simulink model "mcb_pmsm_foc_hall_f28069m"  (R2023b)
settings: Solver=FixedStepDiscrete  StartTime=0.0  StopTime=8  RelTol=1e-3  EnableMultiTasking=on
InitFcn:
  | mcb_pmsm_foc_hall_f28069m_data;
values from neighbouring files (symbols this model uses):
  inverter = mcb_SetInverterParameters('DRV8312-C2-KIT')    [mcb_pmsm_foc_hall_f28069m_data.m]    (also in mcb_pmsm_foc_hall_f28379d_data.m = mcb_updateInverterParameters(pmsm,inverter,target))
  PI_params = mcb_SetControllerParameters(pmsm,inverter,PU_System,T_pwm,Ts,Ts_speed)    [mcb_pmsm_foc_hall_f28069m_data.m]    (also in mcb_pmsm_foc_hall_f28379d_data.m)
  pmsm = mcb_SetPMSMMotorParameters('BLY171D')    [mcb_pmsm_foc_hall_f28069m_data.m]    (also in mcb_pmsm_foc_hall_f28379d_data.m = mcb_SetPMSMMotorParameters("custom"))
  target = mcb_SetProcessorDetails('F28069M',PWM_frequency)    [mcb_pmsm_foc_hall_f28069m_data.m]    (also in mcb_pmsm_foc_hall_f28379d_data.m = mcb_SetProcessorDetails('F28379D',PWM_frequency))
  Ts = T_pwm    (= 5e-05)    [mcb_pmsm_foc_hall_f28069m_data.m]    (also in mcb_pmsm_foc_hall_f28379d_data.m = 6.25e-05)
  Ts_motor = T_pwm/2    (= 2.5e-05)    [mcb_pmsm_foc_hall_f28069m_data.m]    (also in mcb_pmsm_foc_hall_f28379d_data.m = 3.125e-05)
  Ts_simulink = T_pwm/2    (= 2.5e-05)    [mcb_pmsm_foc_hall_f28069m_data.m]    (also in mcb_pmsm_foc_hall_f28379d_data.m = 3.125e-05)
  Ts_speed = 10*Ts    (= 0.0005)    [mcb_pmsm_foc_hall_f28069m_data.m]    (also in mcb_pmsm_foc_hall_f28379d_data.m = 0.000625)
undefined symbols (not defined in the file or in its folder): Down, GPTRIP1SEL, GPTRIP2SEL, TZ1, TZ2, Up
libraries: simulink x14, mcbcontrolslib x9, mcbpositiondecoderlib x7, idelinklib_common x6, c2802xlib x5, c280xlib x5, svdschedulerlib x5, slpidlib x3, c2806xlib x3, svdutilitieslib x2, mcbplantlib x1, autolibpmsmexterior x1
(part 1 of 3)
settings Model: Creator=The MathWorks, Inc.  LastModifiedBy=The MathWorks, Inc.
settings SolverCC: AlgebraicLoopSolver=TrustRegion  AutoInsertRateTranBlk=on
settings DataIOCC: LimitDataPoints=on  SaveFormat=Array  SaveOutput=off  SaveTime=off  ReturnWorkspaceOutputs=off
settings OptimizationCC: DefaultParameterBehavior=Inlined  InlineInvariantSignals=on  OptimizeBlockIOStorage=off  BufferReuse=off  ReuseModelBlockBuffer=off  GlobalBufferReuse=off  ExpressionFolding=off  ExpressionDepthLimit=2147483647  LocalBlockOutputs=off  InitFltsAndDblsToZero=on  NoFixptDivByZeroProtection=on  EfficientFloat2IntCast=on  EfficientMapNaN2IntZero=off  LifeSpan=inf  MaxStackSize=64  OptimizeDataStoreBuffers=off  BusAssignmentInplaceUpdate=off  EfficientTunableParamExpr=on
settings DebuggingCC: AlgebraicLoopMsg=error  ArtificialAlgebraicLoopMsg=error  CheckSSInitialOutputMsg=off  MergeDetectMultiDrivingBlocksExec=none  SolverPrmCheckMsg=warning  InheritedTsInSrcMsg=none  MultiTaskDSMMsg=none  MultiTaskCondExecSysMsg=none  TasksWithSamePriorityMsg=none  SigSpecEnsureSampleTimeMsg=none  ParameterPrecisionLossMsg=none  ParameterTunabilityLossMsg=error  FcnCallInpInsideContextMsg=warning  UnconnectedInputMsg=warning  UnconnectedOutputMsg=warning  UnconnectedLineMsg=warning  AllowSymbolicDim=off  StateNameClashWarn=warning  SFUnexpectedBacktrackingDiag=warning  SFNoUnconditionalDefaultTransitionDiag=warning  SFExecutionAtInitializationDiag=none  ArithmeticOperatorsInVariantConditions=warning
settings HardwareCC: ProdBitPerChar=16  ProdBitPerInt=16  ProdBitPerPointer=32  ProdBitPerSizeT=32  ProdBitPerPtrDiffT=32  ProdLargestAtomicInteger=Integer  ProdLargestAtomicFloat=None  ProdWordSize=16  ProdLongLongMode=on  ProdHWDeviceType=Texas Instruments->C2000  TargetBitPerChar=16  TargetBitPerInt=16  TargetBitPerPointer=16  TargetLargestAtomicInteger=Integer  TargetIntDivRoundTo=Zero  TargetEndianess=LittleEndian  TargetWordSize=16  TargetHWDeviceType=Texas Instruments->C2000  ProdEqTarget=off
settings ModelReferenceCC: EnableRefExpFcnMdlSchedulingChecks=on  PropagateSignalLabelsOutOfModel=off
settings SFSimCC: SimUseLocalCustomCode=off  MATLABDynamicMemAlloc=off
settings RTWCC: Description=Embedded Coder  SystemTargetFile=ert.tlc  HardwareBoard=TI Piccolo F2806x  TemplateMakefile=ert_default_tmf  PostCodeGenCommand=; codertarget.postCodeGenHookCommand(h)  GenerateReport=on  RTWUseLocalCustomCode=off  Toolchain=Texas Instruments Code Composer Studio (C2000)  IncludeHyperlinkInReport=on  GenerateTraceInfo=on  GenerateTraceReport=on  GenerateTraceReportSl=on  GenerateTraceReportSf=on  GenerateTraceReportEml=on  DLArmComputeVersion=19.05
settings CodeAppCC: IgnoreCustomStorageClasses=off  CustomSymbolStrType=$N$R$M  StateflowObjectComments=on  InternalIdentifier=Classic
settings ERTTargetCC: TargetFcnLib=ansi_tfl_tmw_new.mat  CodeReplacementLibrary=TI C28x  MultiwordLength=2048  ParMdlRefBuildCompliant=off  CompOptLevelCompliant=off  ConcurrentExecutionCompliant=off  CPPClassGenCompliant=off  ExtModeStaticAllocSize=2048  ExtModeMexFile=TIC2000ExternalModeOpen  ExtModeIntrfLevel=Level2 - Open  InlinedParameterPlacement=NonHierarchical  ConvertIfToSwitch=off  SuppressUnreachableDefaultCases=off  MemSecPackage=tic2000demospkg
settings ConfigComp: CovMetricSettings=dw  CovSaveCumulativeToWorkspaceVar=on  CovSaveSingleToWorkspaceVar=on  CovExternalEMLEnable=off  CovSFcnEnable=off

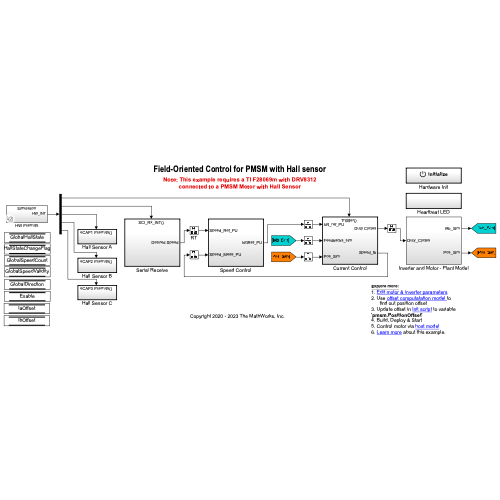
[thumbnail: Simulink's stored preview of the top-level diagram]
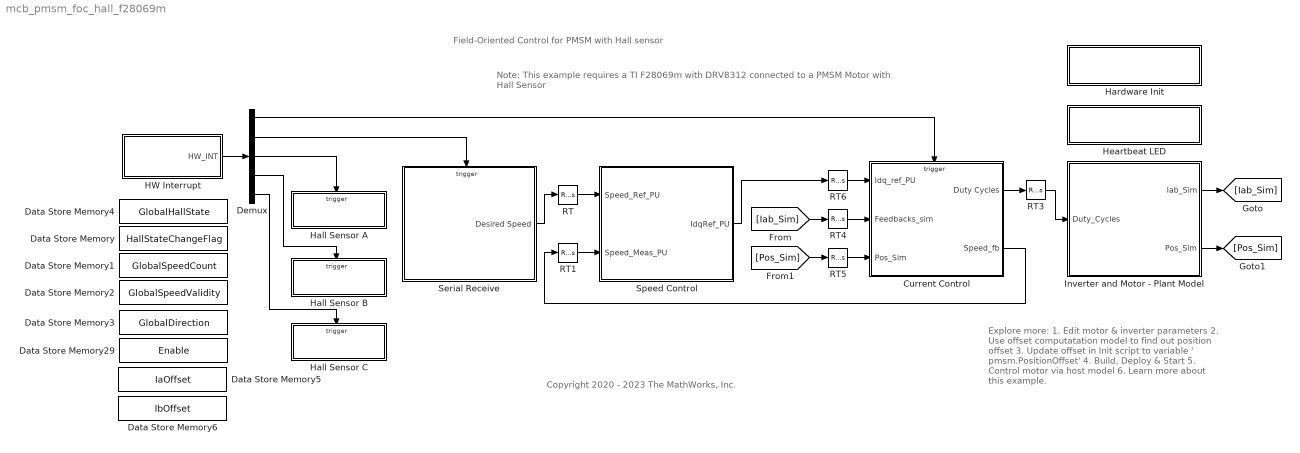
== system mcb_pmsm_foc_hall_f28069m ==
  note: Copyright 2020 - 2023 The MathWorks, Inc.
  note: Field-Oriented Control for PMSM with Hall sensor
  note: Note: This example requires a TI F28069m with DRV8312
      | connected to a PMSM Motor with Hall Sensor
  note: Explore more:
      | 1. Edit motor & inverter parameters
      | 2. Use offset computatation model to
      | find out position offset
      | 3. Update offset in Init script to variable ' pmsm.PositionOffset'
      | 4. Build, Deploy & Start
      | 5. Control motor via host model
      | 6. Learn more about this example.
  Current Control : Subsystem
      settings: RTWSystemCode=Nonreusable function
  Data Store Memory : DataStoreMemory  DataStoreName=HallStateChangeFlag  ShowAdditionalParam=off
  Data Store Memory1 : DataStoreMemory  DataStoreName=GlobalSpeedCount  ShowAdditionalParam=off
  Data Store Memory2 : DataStoreMemory  DataStoreName=GlobalSpeedValidity  ShowAdditionalParam=off
  Data Store Memory29 : DataStoreMemory  DataStoreName=Enable  InitialValue=1  ShowAdditionalParam=off  OutDataTypeStr=boolean
  Data Store Memory3 : DataStoreMemory  DataStoreName=GlobalDirection  ShowAdditionalParam=off
  Data Store Memory4 : DataStoreMemory  DataStoreName=GlobalHallState  ShowAdditionalParam=off  OutDataTypeStr=uint32
  Data Store Memory5 : DataStoreMemory  DataStoreName=IaOffset  InitialValue=inverter.CtSensAOffset  ShowAdditionalParam=off
  Data Store Memory6 : DataStoreMemory  DataStoreName=IbOffset  InitialValue=inverter.CtSensBOffset  ShowAdditionalParam=off
  Demux : Demux  Outputs=5
  HW Interrupt : Subsystem  Variant=on  VariantControlMode=sim codegen switching
  Hall Sensor A : Subsystem
  Hall Sensor B : Subsystem
  Hall Sensor C : Subsystem
  Hardware Init : Subsystem  TreatAsAtomicUnit=on
  Heartbeat LED : Subsystem  TreatAsAtomicUnit=on
  Inverter and Motor - Plant Model : Subsystem
  RT{,3..6} (5 alike) : RateTransition  Deterministic=off
  RT1 : RateTransition  Deterministic=off  OutPortSampleTime=Ts_speed
  Serial Receive : Subsystem  SystemSampleTime=1e-3
  Speed Control : Subsystem  TreatAsAtomicUnit=on  SystemSampleTime=Ts_speed
  wires:
  [Iab_Sim] -> RT4/1
  RT1/1 -> Speed Control/2(Speed_Meas_PU)
  [Pos_Sim] -> RT5/1
  Speed Control/1(IdqRef_PU) -> RT6/1
  Inverter and Motor - Plant Model/1(Iab_Sim) -> [Iab_Sim]
  RT/1 -> Speed Control/1(Speed_Ref_PU)
  Demux/3 -> Hall Sensor A/Trigger
  Demux/5 -> Hall Sensor C/Trigger
  RT6/1 -> Current Control/1(Idq_ref_PU)
  HW Interrupt/1(HW_INT) -> Demux/1
  Demux/1 -> Current Control/Trigger
  RT3/1 -> Inverter and Motor - Plant Model/1(Duty_Cycles)
  Demux/2 -> Serial Receive/Trigger
  RT4/1 -> Current Control/2(Feedbacks_sim)
  Serial Receive/1(Desired Speed) -> RT/1
  Current Control/1(Duty Cycles) -> RT3/1
  Inverter and Motor - Plant Model/2(Pos_Sim) -> [Pos_Sim]
  Demux/4 -> Hall Sensor B/Trigger
  RT5/1 -> Current Control/3(Pos_Sim)
  Current Control/2(Speed_fb) -> RT1/1

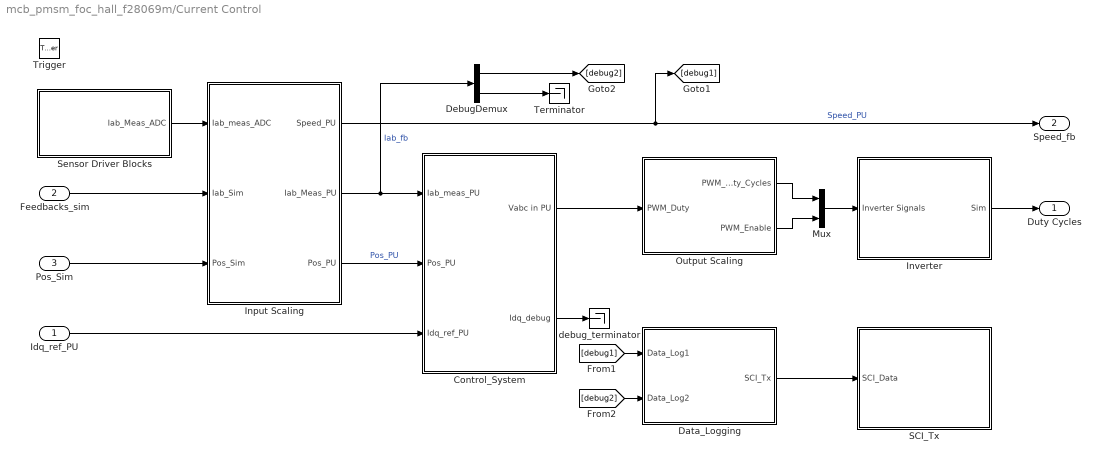
== system mcb_pmsm_foc_hall_f28069m/Current Control ==
  Idq_ref_PU : Inport
  Feedbacks_sim : Inport  Port=2
  Pos_Sim : Inport  Port=3
  Trigger : TriggerPort  TriggerType=function-call  VariantControl=Variant
  Control_System : Subsystem
  Data_Logging : Subsystem
  DebugDemux : Demux  Outputs=2
  Input Scaling : Subsystem  Variant=on  VariantControlMode=sim codegen switching  VariantControl=Variant1  PropagateVariantConditions=on
  Inverter : Subsystem  Variant=on  VariantControlMode=sim codegen switching
  Mux : Mux  Inputs=2
  Output Scaling : Subsystem
  SCI_Tx : Subsystem  Variant=on  VariantControlMode=sim codegen switching
  Sensor Driver Blocks : Subsystem  Variant=on  VariantControlMode=sim codegen switching
  Terminator : Terminator
  debug_terminator : Terminator
  Duty Cycles : Outport  InitialOutput=0  VectorParamsAs1DForOutWhenUnconnected=off
  Speed_fb : Outport  Port=2  InitialOutput=0  VectorParamsAs1DForOutWhenUnconnected=off
  wires:
  Sensor Driver Blocks/1(Iab_Meas_ADC) -> Input Scaling/1(Iab_meas_ADC)
  Control_System/1(Vabc in PU) -> Output Scaling/1(PWM_Duty)
  Input Scaling/3(Pos_PU) -> Control_System/2(Pos_PU)  "Pos_PU"
  Idq_ref_PU/1 -> Control_System/3(Idq_ref_PU)
  Input Scaling/2(Iab_Meas_PU) -> DebugDemux/1, Control_System/1(Iab_meas_PU)  "Iab_fb"
  Input Scaling/1(Speed_PU) -> [debug1], Speed_fb/1  "Speed_PU"
  Pos_Sim/1 -> Input Scaling/3(Pos_Sim)
  Feedbacks_sim/1 -> Input Scaling/2(Iab_Sim)
  Mux/1 -> Inverter/1(Inverter Signals)
  Output Scaling/1(PWM_Duty_Cycles) -> Mux/1
  Output Scaling/2(PWM_Enable) -> Mux/2
  Inverter/1(Sim) -> Duty Cycles/1
  [debug2] -> Data_Logging/2(Data_Log2)
  [debug1] -> Data_Logging/1(Data_Log1)
  DebugDemux/1 -> [debug2]
  DebugDemux/2 -> Terminator/1
  Control_System/2(Idq_debug) -> debug_terminator/1
  Data_Logging/1(SCI_Tx) -> SCI_Tx/1(SCI_Data)

== system mcb_pmsm_foc_hall_f28069m/HW Interrupt ==
  Code Generation : Subsystem  VariantControl=(codegen)
  Simulation : Subsystem  VariantControl=(sim)
  HW_INT : Outport  VectorParamsAs1DForOutWhenUnconnected=off  OutputFunctionCall=on

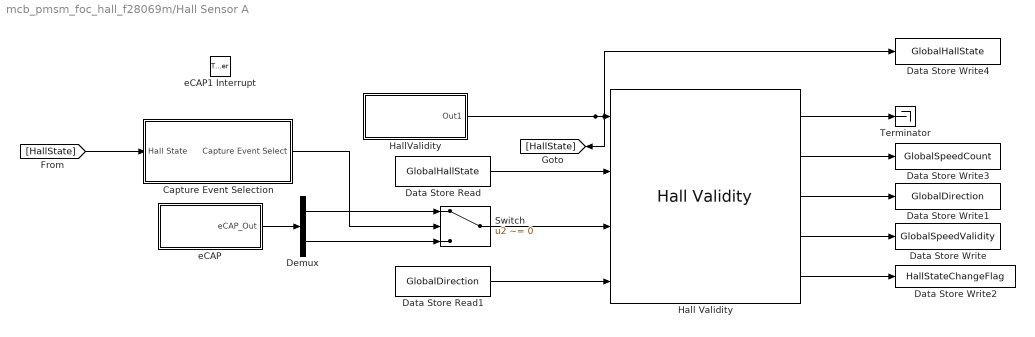
== system mcb_pmsm_foc_hall_f28069m/Hall Sensor A ==
  eCAP1 Interrupt : TriggerPort  TriggerType=function-call  VariantControl=Variant
  Capture Event Selection : Subsystem
  Data Store Read : DataStoreRead  Priority=1  DataStoreName=GlobalHallState  IndexOptions=Index vector (dialog)  Indices=1  OutputSizes=1
  Data Store Read1 : DataStoreRead  DataStoreName=GlobalDirection  IndexOptions=Index vector (dialog)  Indices=1  OutputSizes=1
  Data Store Write : DataStoreWrite  DataStoreName=GlobalSpeedValidity  IndexOptions=Index vector (dialog)  Indices=1  OutputSizes=1
  Data Store Write1 : DataStoreWrite  DataStoreName=GlobalDirection  IndexOptions=Index vector (dialog)  Indices=1  OutputSizes=1
  Data Store Write2 : DataStoreWrite  DataStoreName=HallStateChangeFlag  IndexOptions=Index vector (dialog)  Indices=1  OutputSizes=1
  Data Store Write3 : DataStoreWrite  DataStoreName=GlobalSpeedCount  IndexOptions=Index vector (dialog)  Indices=1  OutputSizes=1
  Data Store Write4 : DataStoreWrite  Priority=2  DataStoreName=GlobalHallState  IndexOptions=Index vector (dialog)  Indices=1  OutputSizes=1
  Demux : Demux  Outputs=2
  Hall Validity : mcbpositiondecoderlib/Hall Validity  hallSequence=ABC  sequence=[5,4,6,2,3,1]  CounterSize=32 bits
  HallValidity : Subsystem  Variant=on  VariantControlMode=sim codegen switching
  Switch : Switch  Criteria=u2 ~= 0  SaturateOnIntegerOverflow=off  InputSameDT=off
  Terminator : Terminator
  eCAP : Subsystem  Variant=on  VariantControlMode=sim codegen switching
  wires:
  Hall Validity/3 -> Data Store Write1/1
  Hall Validity/5 -> Data Store Write2/1
  Hall Validity/4 -> Data Store Write/1
  Data Store Read/1 -> Hall Validity/2
  Data Store Read1/1 -> Hall Validity/4
  Switch/1 -> Hall Validity/3
  Hall Validity/2 -> Data Store Write3/1
  Demux/2 -> Switch/3
  Demux/1 -> Switch/1
  Hall Validity/1 -> Terminator/1
  Capture Event Selection/1(Capture Event Select) -> Switch/2
  [HallState] -> Capture Event Selection/1(Hall State)
  eCAP/1(eCAP_Out) -> Demux/1
  HallValidity/1(Out1) -> [HallState], Data Store Write4/1, Hall Validity/1

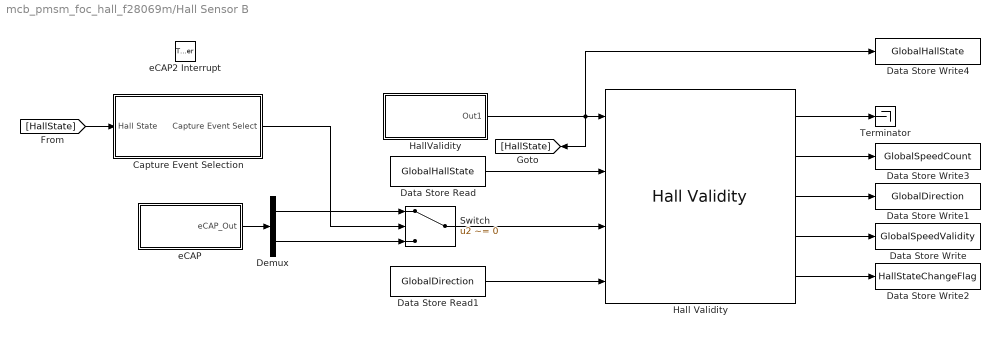
== system mcb_pmsm_foc_hall_f28069m/Hall Sensor B ==
  eCAP2 Interrupt : TriggerPort  TriggerType=function-call  VariantControl=Variant
  Capture Event Selection : Subsystem
  Data Store Read : DataStoreRead  Priority=1  DataStoreName=GlobalHallState  IndexOptions=Index vector (dialog)  Indices=1  OutputSizes=1
  Data Store Read1 : DataStoreRead  DataStoreName=GlobalDirection  IndexOptions=Index vector (dialog)  Indices=1  OutputSizes=1
  Data Store Write : DataStoreWrite  DataStoreName=GlobalSpeedValidity  IndexOptions=Index vector (dialog)  Indices=1  OutputSizes=1
  Data Store Write1 : DataStoreWrite  DataStoreName=GlobalDirection  IndexOptions=Index vector (dialog)  Indices=1  OutputSizes=1
  Data Store Write2 : DataStoreWrite  DataStoreName=HallStateChangeFlag  IndexOptions=Index vector (dialog)  Indices=1  OutputSizes=1
  Data Store Write3 : DataStoreWrite  DataStoreName=GlobalSpeedCount  IndexOptions=Index vector (dialog)  Indices=1  OutputSizes=1
  Data Store Write4 : DataStoreWrite  Priority=2  DataStoreName=GlobalHallState  IndexOptions=Index vector (dialog)  Indices=1  OutputSizes=1
  Demux : Demux  Outputs=2
  Hall Validity : mcbpositiondecoderlib/Hall Validity  hallSequence=ABC  sequence=[5,4,6,2,3,1]  CounterSize=32 bits
  HallValidity : Subsystem  Variant=on  VariantControlMode=sim codegen switching
  Switch : Switch  Criteria=u2 ~= 0  Threshold=3  SaturateOnIntegerOverflow=off  InputSameDT=off
  Terminator : Terminator
  eCAP : Subsystem  Variant=on  VariantControlMode=sim codegen switching
  wires:
  Hall Validity/3 -> Data Store Write1/1
  Hall Validity/5 -> Data Store Write2/1
  Hall Validity/4 -> Data Store Write/1
  Data Store Read1/1 -> Hall Validity/4
  Hall Validity/2 -> Data Store Write3/1
  Data Store Read/1 -> Hall Validity/2
  Demux/1 -> Switch/1
  Demux/2 -> Switch/3
  eCAP/1(eCAP_Out) -> Demux/1
  Switch/1 -> Hall Validity/3
  Hall Validity/1 -> Terminator/1
  [HallState] -> Capture Event Selection/1(Hall State)
  Capture Event Selection/1(Capture Event Select) -> Switch/2
  HallValidity/1(Out1) -> Data Store Write4/1, Hall Validity/1, [HallState]

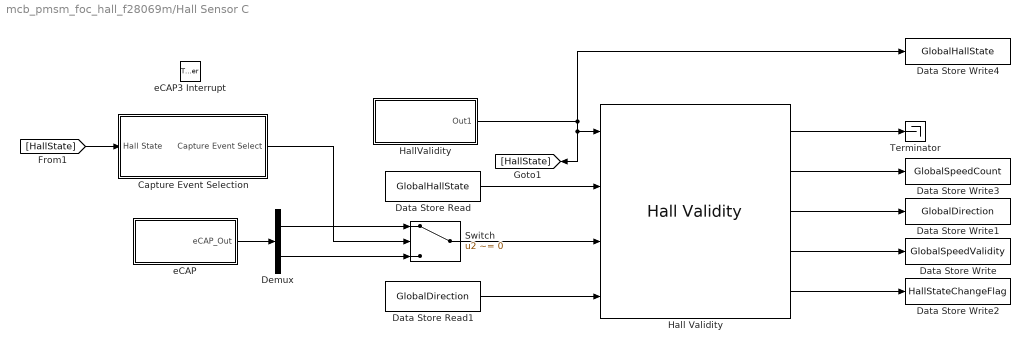
== system mcb_pmsm_foc_hall_f28069m/Hall Sensor C ==
  eCAP3 Interrupt : TriggerPort  TriggerType=function-call  VariantControl=Variant
  Capture Event Selection : Subsystem
  Data Store Read : DataStoreRead  Priority=1  DataStoreName=GlobalHallState  IndexOptions=Index vector (dialog)  Indices=1  OutputSizes=1
  Data Store Read1 : DataStoreRead  DataStoreName=GlobalDirection  IndexOptions=Index vector (dialog)  Indices=1  OutputSizes=1
  Data Store Write : DataStoreWrite  DataStoreName=GlobalSpeedValidity  IndexOptions=Index vector (dialog)  Indices=1  OutputSizes=1
  Data Store Write1 : DataStoreWrite  DataStoreName=GlobalDirection  IndexOptions=Index vector (dialog)  Indices=1  OutputSizes=1
  Data Store Write2 : DataStoreWrite  DataStoreName=HallStateChangeFlag  IndexOptions=Index vector (dialog)  Indices=1  OutputSizes=1
  Data Store Write3 : DataStoreWrite  DataStoreName=GlobalSpeedCount  IndexOptions=Index vector (dialog)  Indices=1  OutputSizes=1
  Data Store Write4 : DataStoreWrite  Priority=2  DataStoreName=GlobalHallState  IndexOptions=Index vector (dialog)  Indices=1  OutputSizes=1
  Demux : Demux  Outputs=2
  Hall Validity : mcbpositiondecoderlib/Hall Validity  hallSequence=ABC  sequence=[5,4,6,2,3,1]  CounterSize=32 bits
  HallValidity : Subsystem  Variant=on  VariantControlMode=sim codegen switching
  Switch : Switch  Criteria=u2 ~= 0  Threshold=3  SaturateOnIntegerOverflow=off  InputSameDT=off
  Terminator : Terminator
  eCAP : Subsystem  Variant=on  VariantControlMode=sim codegen switching
  wires:
  Hall Validity/3 -> Data Store Write1/1
  Hall Validity/5 -> Data Store Write2/1
  Hall Validity/4 -> Data Store Write/1
  Data Store Read1/1 -> Hall Validity/4
  Hall Validity/2 -> Data Store Write3/1
  Data Store Read/1 -> Hall Validity/2
  Demux/1 -> Switch/1
  Demux/2 -> Switch/3
  eCAP/1(eCAP_Out) -> Demux/1
  Switch/1 -> Hall Validity/3
  Hall Validity/1 -> Terminator/1
  [HallState] -> Capture Event Selection/1(Hall State)
  Capture Event Selection/1(Capture Event Select) -> Switch/2
  HallValidity/1(Out1) -> [HallState], Hall Validity/1, Data Store Write4/1

== system mcb_pmsm_foc_hall_f28069m/Hardware Init ==
  Constant : Constant
  Event Listener : EventListener  DisableCoverage=on  EventName=reset
  Variant Subsystem : Subsystem  Variant=on  VariantControlMode=sim codegen switching
  wires:
  Constant/1 -> Variant Subsystem/1(Input)

== system mcb_pmsm_foc_hall_f28069m/Heartbeat LED ==
  note: Heartbeat LED 1HZ
  Heartbeat LED : Subsystem  Variant=on  VariantControlMode=sim codegen switching
  RED_LED : Constant  OutDataTypeStr=uint16  SampleTime=0.5
  wires:
  RED_LED/1 -> Heartbeat LED/1(In1)

== system mcb_pmsm_foc_hall_f28069m/Inverter and Motor - Plant Model ==
  Duty_Cycles : Inport
  Codegeneration : Subsystem
  Simulation : Subsystem
  Variant Sink : VariantSink  VariantControlMode=sim codegen switching
  Variant Source : VariantSource  VariantControlMode=sim codegen switching
  Variant Source1 : VariantSource  VariantControlMode=sim codegen switching
  Iab_Sim : Outport  VectorParamsAs1DForOutWhenUnconnected=off
  Pos_Sim : Outport  Port=2  VectorParamsAs1DForOutWhenUnconnected=off
  wires:
  Duty_Cycles/1 -> Variant Sink/1
  Variant Source/1 -> Iab_Sim/1
  Variant Source1/1 -> Pos_Sim/1
  Codegeneration/1(Iab_fb_Sim) -> Variant Source/1
  Codegeneration/2(Pos_fb_Sim) -> Variant Source1/1
  Variant Sink/1 -> Codegeneration/1(Duty_Cycles)
  Variant Sink/2 -> Simulation/1(Duty_Cycles)
  Simulation/1(Iab_fb_Sim) -> Variant Source/2
  Simulation/2(Pos_fb_Sim) -> Variant Source1/2

== system mcb_pmsm_foc_hall_f28069m/Serial Receive ==
  SCI_Rx_INT : TriggerPort  TriggerType=function-call  VariantControl=Variant
  Data Store Write : DataStoreWrite  DataStoreName=Enable  IndexOptions=Index vector (dialog)  Indices=1  OutputSizes=1
  Data Type Conversion1 : DataTypeConversion  OutDataTypeStr=dataType  RndMeth=Simplest  SaturateOnIntegerOverflow=off
  Data Type Conversion3 : DataTypeConversion  OutDataTypeStr=boolean  RndMeth=Simplest  SaturateOnIntegerOverflow=off
  Data_Conditioning : Subsystem
  Demux : Demux  Outputs=2
  SCI_Rx : Subsystem  Variant=on  VariantControlMode=sim codegen switching
  Desired Speed : Outport  VectorParamsAs1DForOutWhenUnconnected=off
  wires:
  Data_Conditioning/1(Out1) -> Demux/1
  Demux/1 -> Data Type Conversion1/1
  Data Type Conversion3/1 -> Data Store Write/1
  Demux/2 -> Data Type Conversion3/1
  SCI_Rx/1(Data) -> Data_Conditioning/1(In1)
  Data Type Conversion1/1 -> Desired Speed/1

== system mcb_pmsm_foc_hall_f28069m/Speed Control ==
  Speed_Ref_PU : Inport
  Speed_Meas_PU : Inport  Port=2
  Id_ref : Constant  Value=0  OutDataTypeStr=dataType  SampleTime=Ts_speed
  Mux1 : Mux  Inputs=2
  PI_Controller_Speed : Subsystem
  Speed_Ref_Selector : Subsystem
  IdqRef_PU : Outport  VectorParamsAs1DForOutWhenUnconnected=off
  wires:
  Speed_Meas_PU/1 -> Speed_Ref_Selector/2(Speed_Ref_Open), PI_Controller_Speed/2(N_fb)  "Speed_fb"
  Id_ref/1 -> Mux1/1
  PI_Controller_Speed/1(Iq_ref) -> Mux1/2
  Mux1/1 -> IdqRef_PU/1
  Speed_Ref_PU/1 -> Speed_Ref_Selector/1(Speed_Ref_In)
  Speed_Ref_Selector/1(Speed_Ref_PU) -> PI_Controller_Speed/1(N_ref)  "Speed_Ref"

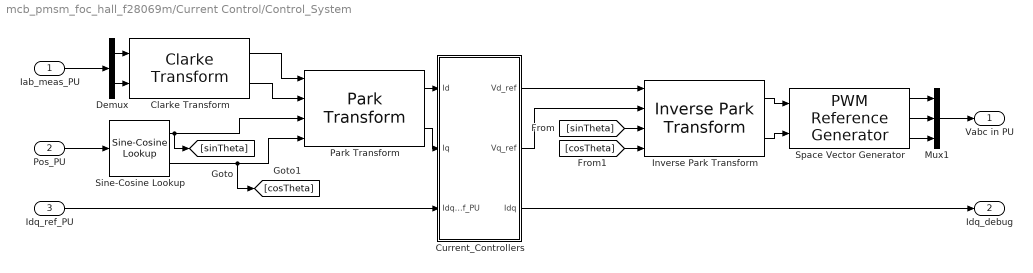
== system mcb_pmsm_foc_hall_f28069m/Current Control/Control_System ==
  Iab_meas_PU : Inport
  Pos_PU : Inport  Port=2
  Idq_ref_PU : Inport  Port=3
  Clarke Transform : mcbcontrolslib/Clarke Transform  VariantControl=Variant2  PhaseInput=Two inputs  EnPowerInv=off
  Current_Controllers : Subsystem
  Demux : Demux  Outputs=2
  Inverse Park Transform : mcbcontrolslib/Inverse Park Transform  PhaseInput=Two inputs  AxisAlignment=D-axis  ThetaInput=Sine and Cosine electrical position  AngleInput=Per-unit  N_points=1024
  Mux1 : Mux  Inputs=3
  Park Transform : mcbcontrolslib/Park Transform  PhaseInput=Two inputs  AxisAlignment=D-axis  ThetaInput=Sine and Cosine electrical position  AngleInput=Per-unit  N_points=1024
  Sine-Cosine Lookup : mcbcontrolslib/Sine-Cosine Lookup  AngleInput=Per-unit  N_points=1024
  Space Vector Generator : mcbcontrolslib/PWM Reference Generator  inSignal=Valphabeta  modType=SVM: space vector modulation
  Vabc in PU : Outport  VectorParamsAs1DForOutWhenUnconnected=off
  Idq_debug : Outport  Port=2  VectorParamsAs1DForOutWhenUnconnected=off
  wires:
  Mux1/1 -> Vabc in PU/1
  Current_Controllers/1(Vd_ref) -> Inverse Park Transform/1
  Pos_PU/1 -> Sine-Cosine Lookup/1
  [sinTheta] -> Inverse Park Transform/3
  Inverse Park Transform/2 -> Space Vector Generator/2
  Space Vector Generator/3 -> Mux1/3
  Clarke Transform/2 -> Park Transform/2
  Space Vector Generator/1 -> Mux1/1
  Space Vector Generator/2 -> Mux1/2
  Current_Controllers/2(Vq_ref) -> Inverse Park Transform/2
  Idq_ref_PU/1 -> Current_Controllers/3(Idq_ref_PU)
  Iab_meas_PU/1 -> Demux/1
  Sine-Cosine Lookup/2 -> [cosTheta], Park Transform/4
  Clarke Transform/1 -> Park Transform/1
  Sine-Cosine Lookup/1 -> Park Transform/3, [sinTheta]
  Demux/1 -> Clarke Transform/1
  Demux/2 -> Clarke Transform/2
  Inverse Park Transform/1 -> Space Vector Generator/1
  Park Transform/2 -> Current_Controllers/2(Iq)
  Park Transform/1 -> Current_Controllers/1(Id)
  [cosTheta] -> Inverse Park Transform/4
  Current_Controllers/3(Idq) -> Idq_debug/1

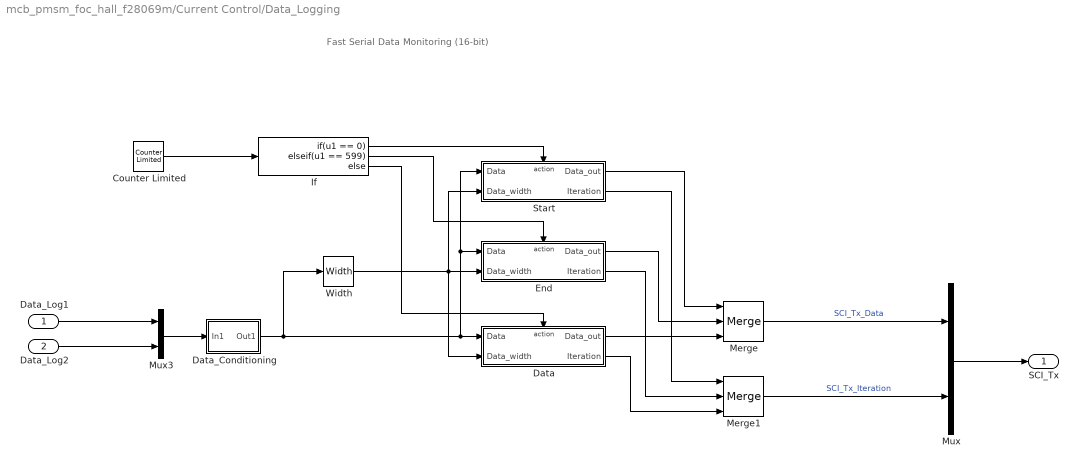
== system mcb_pmsm_foc_hall_f28069m/Current Control/Data_Logging ==
  note: Fast Serial Data Monitoring (16-bit)
  Data_Log1 : Inport
  Data_Log2 : Inport  Port=2
  Counter Limited : simulink/Sources/Counter Limited  uplimit=599  tsamp=-1
  Data : Subsystem  TreatAsAtomicUnit=on
  Data_Conditioning : Subsystem
  End : Subsystem  TreatAsAtomicUnit=on
  If : If  IfExpression=u1 == 0  ElseIfExpressions=u1 == 599
  Merge : Merge  Inputs=3
  Merge1 : Merge  Inputs=3
  Mux : Mux  Inputs=2
  Mux3 : Mux  Inputs=2
  Start : Subsystem  TreatAsAtomicUnit=on
  Width : Width  OutDataTypeMode=All ports same datatype  DataType=uint16
  SCI_Tx : Outport
  wires:
  If/3 -> Data/Action
  Data/1(Data_out) -> Merge/3
  Width/1 -> Data/2(Data_width), End/2(Data_width), Start/2(Data_width)
  Merge/1 -> Mux/1  "SCI_Tx_Data"
  Counter Limited/1 -> If/1
  Start/2(Iteration) -> Merge1/1
  Start/1(Data_out) -> Merge/1
  If/2 -> End/Action
  Merge1/1 -> Mux/2  "SCI_Tx_Iteration"
  If/1 -> Start/Action
  End/1(Data_out) -> Merge/2
  End/2(Iteration) -> Merge1/2
  Data/2(Iteration) -> Merge1/3
  Data_Log1/1 -> Mux3/1
  Data_Conditioning/1(Out1) -> Width/1, Data/1(Data), End/1(Data), Start/1(Data)
  Mux/1 -> SCI_Tx/1
  Mux3/1 -> Data_Conditioning/1(In1)
  Data_Log2/1 -> Mux3/2

== system mcb_pmsm_foc_hall_f28069m/Current Control/Input Scaling ==
  Iab_meas_ADC : Inport
  Iab_Sim : Inport  Port=2
  Pos_Sim : Inport  Port=3
  Read_Sensor (codegen) : Subsystem  VariantControl=(codegen)
  Read_Sensor (sim) : Subsystem  VariantControl=(sim)
  Speed_PU : Outport  VectorParamsAs1DForOutWhenUnconnected=off
  Iab_Meas_PU : Outport  Port=2  VectorParamsAs1DForOutWhenUnconnected=off
  Pos_PU : Outport  Port=3  VectorParamsAs1DForOutWhenUnconnected=off

== system mcb_pmsm_foc_hall_f28069m/Current Control/Inverter ==
  Inverter Signals : Inport
  Code Generation : Subsystem  VariantControl=(codegen)
  Simulation : Subsystem  VariantControl=(sim)
  Sim : Outport  VectorParamsAs1DForOutWhenUnconnected=off

== system mcb_pmsm_foc_hall_f28069m/Current Control/Output Scaling ==
  PWM_Duty : Inport
  Constant : Constant  Value=0.5  OutDataTypeStr=dataType  SampleTime=-1
  Data Type Conversion : DataTypeConversion  OutDataTypeStr=dataType  SaturateOnIntegerOverflow=off  RndMeth=Floor
  Enable : DataStoreRead  DataStoreName=Enable  IndexOptions=Index vector (dialog)  Indices=1  OutputSizes=1
  One_by_Two : Gain  Gain=0.5  RndMeth=Simplest  OutDataTypeStr=Inherit: Same as input
  Sum : Sum  Inputs=|++
  PWM_Duty_Cycles : Outport
  PWM_Enable : Outport  Port=2
  wires:
  PWM_Duty/1 -> One_by_Two/1
  Constant/1 -> Sum/2
  One_by_Two/1 -> Sum/1
  Sum/1 -> PWM_Duty_Cycles/1  "PWM_Duty_Cycles"
  Enable/1 -> Data Type Conversion/1  "PWM_En"
  Data Type Conversion/1 -> PWM_Enable/1

== system mcb_pmsm_foc_hall_f28069m/Current Control/SCI_Tx ==
  SCI_Data : Inport
  Code Generation : Subsystem  VariantControl=(codegen)
  Simulation : Subsystem  VariantControl=(sim)

== system mcb_pmsm_foc_hall_f28069m/Current Control/Sensor Driver Blocks ==
  Sensor Driver Blocks (codegen) : Subsystem  VariantControl=(codegen)
  Sensor Driver Blocks (sim) : Subsystem  VariantControl=(sim)
  Iab_Meas_ADC : Outport

== system mcb_pmsm_foc_hall_f28069m/HW Interrupt/Code Generation ==
  HWI_ADCINT1 : svdschedulerlib/Hardware Interrupt v2  ISRGroup=ADC - Analog to Digital Converter  ISRName=ADCA1_INT  ISRNumber=32  NumEventsToServe=1  EventsList={'on','EOC event','1';'off','Overflow event','2';'off','Custom event','3'}  SelectedEvents={'event1'}  TaskPriority=30  DisablePreemption=off  ClearInterruptFlagsAtEndOfEvent=on  InterruptDefinitionFile=$(TARGET_ROOT)/registry/interrupts/F2837xS_interrupts.xml  HardwareBoard=F2837x  EnableSimPort=off
      settings: LibrarySourceBlock=c2000lib/Scheduling/Hardware Interrupt
  HWI_ECAP1_INT : svdschedulerlib/Hardware Interrupt v2  ISRGroup=ADC - Analog to Digital Converter  ISRName=ADCA1_INT  ISRNumber=32  NumEventsToServe=1  EventsList={'on','EOC event','1';'off','Overflow event','2';'off','Custom event','3'}  SelectedEvents={'event1'}  TaskPriority=25  DisablePreemption=on  ClearInterruptFlagsAtEndOfEvent=on  InterruptDefinitionFile=$(TARGET_ROOT)/registry/interrupts/F2837xS_interrupts.xml  HardwareBoard=F2837x  EnableSimPort=off
      settings: LibrarySourceBlock=c2000lib/Scheduling/Hardware Interrupt
  HWI_ECAP2_INT : svdschedulerlib/Hardware Interrupt v2  ISRGroup=ADC - Analog to Digital Converter  ISRName=ADCA1_INT  ISRNumber=32  NumEventsToServe=1  EventsList={'on','EOC event','1';'off','Overflow event','2';'off','Custom event','3'}  SelectedEvents={'event1'}  TaskPriority=25  DisablePreemption=on  ClearInterruptFlagsAtEndOfEvent=on  InterruptDefinitionFile=$(TARGET_ROOT)/registry/interrupts/F2837xS_interrupts.xml  HardwareBoard=F2837x  EnableSimPort=off
      settings: LibrarySourceBlock=c2000lib/Scheduling/Hardware Interrupt
  HWI_ECAP3_INT : svdschedulerlib/Hardware Interrupt v2  ISRGroup=ADC - Analog to Digital Converter  ISRName=ADCA1_INT  ISRNumber=32  NumEventsToServe=1  EventsList={'on','EOC event','1';'off','Overflow event','2';'off','Custom event','3'}  SelectedEvents={'event1'}  TaskPriority=25  DisablePreemption=on  ClearInterruptFlagsAtEndOfEvent=on  InterruptDefinitionFile=$(TARGET_ROOT)/registry/interrupts/F2837xS_interrupts.xml  HardwareBoard=F2837x  EnableSimPort=off
      settings: LibrarySourceBlock=c2000lib/Scheduling/Hardware Interrupt
  HWI_SCIRXINTA : svdschedulerlib/Hardware Interrupt v2  ISRGroup=ADC - Analog to Digital Converter  ISRName=ADCA1_INT  ISRNumber=32  NumEventsToServe=1  EventsList={'on','EOC event','1';'off','Overflow event','2';'off','Custom event','3'}  SelectedEvents={'event1'}  TaskPriority=50  DisablePreemption=on  ClearInterruptFlagsAtEndOfEvent=on  InterruptDefinitionFile=$(TARGET_ROOT)/registry/interrupts/F2837xS_interrupts.xml  HardwareBoard=F2837x  EnableSimPort=off
      settings: LibrarySourceBlock=c2000lib/Scheduling/Hardware Interrupt
  Mux : Mux  Inputs=5
  HW_INT : Outport  VectorParamsAs1DForOutWhenUnconnected=off
  wires:
  HWI_ADCINT1/1 -> Mux/1
  HWI_ECAP3_INT/1 -> Mux/5
  HWI_SCIRXINTA/1 -> Mux/2
  HWI_ECAP1_INT/1 -> Mux/3
  HWI_ECAP2_INT/1 -> Mux/4
  Mux/1 -> HW_INT/1

== system mcb_pmsm_foc_hall_f28069m/HW Interrupt/Simulation ==
  Function-Call Generator{,1..3} (4 alike) : simulink/Ports & Subsystems/Function-Call Generator  sample_time=Ts  numberOfIterations=1  DisallowWideOutput=off
  Mux : Mux  Inputs=5
  SCI_Rx_INT : simulink/Ports & Subsystems/Function-Call Generator  sample_time=0.1  numberOfIterations=1  DisallowWideOutput=off
  HW_INT : Outport
  wires:
  SCI_Rx_INT/1 -> Mux/2
  Function-Call Generator/1 -> Mux/1
  Mux/1 -> HW_INT/1
  Function-Call Generator1/1 -> Mux/3
  Function-Call Generator2/1 -> Mux/4
  Function-Call Generator3/1 -> Mux/5

== system mcb_pmsm_foc_hall_f28069m/Hall Sensor A/Capture Event Selection ==
  Hall State : Inport
  If : If  IfExpression=(u1 == 5 | u1 == 3)
  Merge : Merge
  Output 0 : Subsystem  TreatAsAtomicUnit=on
  Output 1 : Subsystem  TreatAsAtomicUnit=on
  Capture Event Select : Outport
  wires:
  Hall State/1 -> If/1
  Merge/1 -> Capture Event Select/1
  Output 0/1(Out1) -> Merge/2
  If/2 -> Output 0/Action
  If/1 -> Output 1/Action
  Output 1/1(Out1) -> Merge/1

== system mcb_pmsm_foc_hall_f28069m/Hall Sensor A/HallValidity ==
  CodeGen : Subsystem  VariantControl=(codegen)
  Sim : Subsystem  VariantControl=(sim)
  Out1 : Outport

== system mcb_pmsm_foc_hall_f28069m/Hall Sensor A/eCAP ==
  Code generation : Subsystem  VariantControl=(codegen)
  Simulation : Subsystem  VariantControl=(sim)
  eCAP_Out : Outport

== system mcb_pmsm_foc_hall_f28069m/Hall Sensor B/Capture Event Selection ==
  Hall State : Inport
  If : If  IfExpression=(u1 == 3 | u1 == 6)
  Merge : Merge
  Output 0 : Subsystem  TreatAsAtomicUnit=on
  Output 1 : Subsystem  TreatAsAtomicUnit=on
  Capture Event Select : Outport
  wires:
  Output 1/1(Out1) -> Merge/1
  Output 0/1(Out1) -> Merge/2
  If/2 -> Output 0/Action
  If/1 -> Output 1/Action
  Hall State/1 -> If/1
  Merge/1 -> Capture Event Select/1

== system mcb_pmsm_foc_hall_f28069m/Hall Sensor B/HallValidity ==
  CodeGen : Subsystem  VariantControl=(codegen)
  Sim : Subsystem  VariantControl=(sim)
  Out1 : Outport

== system mcb_pmsm_foc_hall_f28069m/Hall Sensor B/eCAP ==
  Code generation : Subsystem  VariantControl=(codegen)
  Simulation : Subsystem  VariantControl=(sim)
  eCAP_Out : Outport

== system mcb_pmsm_foc_hall_f28069m/Hall Sensor C/Capture Event Selection ==
  Hall State : Inport
  If : If  IfExpression=(u1 == 5 | u1 == 6)
  Merge : Merge
  Output 0 : Subsystem  TreatAsAtomicUnit=on
  Output 1 : Subsystem  TreatAsAtomicUnit=on
  Capture Event Select : Outport
  wires:
  Output 1/1(Out1) -> Merge/1
  Output 0/1(Out1) -> Merge/2
  If/2 -> Output 0/Action
  If/1 -> Output 1/Action
  Hall State/1 -> If/1
  Merge/1 -> Capture Event Select/1

== system mcb_pmsm_foc_hall_f28069m/Hall Sensor C/HallValidity ==
  CodeGen : Subsystem  VariantControl=(codegen)
  Sim : Subsystem  VariantControl=(sim)
  Out1 : Outport

== system mcb_pmsm_foc_hall_f28069m/Hall Sensor C/eCAP ==
  Code generation : Subsystem  VariantControl=(codegen)
  Simulation : Subsystem  VariantControl=(sim)
  eCAP_Out : Outport

== system mcb_pmsm_foc_hall_f28069m/Hardware Init/Variant Subsystem ==
  Input : Inport
  Code Generation : Subsystem  VariantControl=(codegen)
  Simulation : Subsystem  VariantControl=(sim)

== system mcb_pmsm_foc_hall_f28069m/Heartbeat LED/Heartbeat LED ==
  In1 : Inport
  Code generation : Subsystem  VariantControl=(codegen)
  Simulation : Subsystem  VariantControl=(sim)

== system mcb_pmsm_foc_hall_f28069m/Inverter and Motor - Plant Model/Codegeneration ==
  Duty_Cycles : Inport
  Ground : Ground
  Ground1 : Ground
  Terminator : Terminator
  Iab_fb_Sim : Outport  VectorParamsAs1DForOutWhenUnconnected=off
  Pos_fb_Sim : Outport  Port=2  VectorParamsAs1DForOutWhenUnconnected=off
  wires:
  Duty_Cycles/1 -> Terminator/1
  Ground/1 -> Iab_fb_Sim/1
  Ground1/1 -> Pos_fb_Sim/1

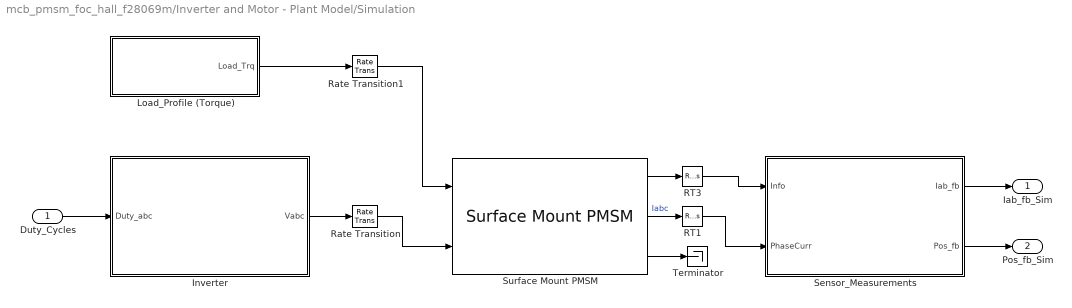
== system mcb_pmsm_foc_hall_f28069m/Inverter and Motor - Plant Model/Simulation ==
  Duty_Cycles : Inport
  Inverter : Subsystem
  Load_Profile (Torque) : Subsystem
  RT1 : RateTransition  Deterministic=off  OutPortSampleTime=Ts_simulink
  RT3 : RateTransition  Deterministic=off  OutPortSampleTime=Ts_simulink
  Rate Transition : RateTransition  Deterministic=off  OutPortSampleTime=Ts_motor
  Rate Transition1 : RateTransition  Deterministic=off  OutPortSampleTime=Ts_motor
  Sensor_Measurements : Subsystem
  Surface Mount PMSM : autolibpmsmexterior/Surface Mount PMSM  port_config=Torque  sim_type=Discrete  Ts=Ts_motor  P=pmsm.p  Rs=pmsm.Rs + inverter.R_board  Ldq_=pmsm.Ld  KConstText=Permanent flux linkage constant (lambda_pm):  lambda_pm=pmsm.FluxPM  Ke=159.9771  Kt=1.323  mechanical=[pmsm.J, pmsm.B, 0]  idq0=[0 0]  theta_init=0  omega_init=0  KConst=pmsm.FluxPM  lambda_pm_calc=pmsm.FluxPM  RefBlkName='autolibpmsmexterior/Surface Mount PMSM'  aMode=5  Ldq="[0.0006      0.0006]"
  Terminator : Terminator
  Iab_fb_Sim : Outport  VectorParamsAs1DForOutWhenUnconnected=off
  Pos_fb_Sim : Outport  Port=2  VectorParamsAs1DForOutWhenUnconnected=off
  wires:
  RT1/1 -> Sensor_Measurements/2(PhaseCurr)
  Surface Mount PMSM/3 -> Terminator/1
  Inverter/1(Vabc) -> Rate Transition/1
  Load_Profile (Torque)/1(Load_Trq) -> Rate Transition1/1
  Surface Mount PMSM/2 -> RT1/1  "Iabc"
  RT3/1 -> Sensor_Measurements/1(Info)
  Surface Mount PMSM/1 -> RT3/1
  Rate Transition1/1 -> Surface Mount PMSM/1
  Rate Transition/1 -> Surface Mount PMSM/2
  Duty_Cycles/1 -> Inverter/1(Duty_abc)
  Sensor_Measurements/1(Iab_fb) -> Iab_fb_Sim/1
  Sensor_Measurements/2(Pos_fb) -> Pos_fb_Sim/1

== system mcb_pmsm_foc_hall_f28069m/Serial Receive/Data_Conditioning ==
  In1 : Inport
  Data Type Conversion1 : DataTypeConversion  OutDataTypeStr=single  RndMeth=Simplest  SaturateOnIntegerOverflow=off
  Data Type Conversion2 : DataTypeConversion  OutDataTypeStr=fixdt(1,16,12)  ConvertRealWorld=Stored Integer (SI)  RndMeth=Simplest  SaturateOnIntegerOverflow=off
  Out1 : Outport  VectorParamsAs1DForOutWhenUnconnected=off
  wires:
  Data Type Conversion1/1 -> Out1/1
  In1/1 -> Data Type Conversion2/1
  Data Type Conversion2/1 -> Data Type Conversion1/1

== system mcb_pmsm_foc_hall_f28069m/Serial Receive/SCI_Rx ==
  Code Generation : Subsystem  VariantControl=(codegen)
  Simulation : Subsystem  VariantControl=(sim)
  Data : Outport

== system mcb_pmsm_foc_hall_f28069m/Speed Control/PI_Controller_Speed ==
  N_ref : Inport
  N_fb : Inport  Port=2
  Data Store Read1 : DataStoreRead  DataStoreName=Enable  IndexOptions=Index vector (dialog)  Indices=1  OutputSizes=1
  Discrete PI Controller with anti-windup & reset : slpidlib/PID Controller  Controller=PI  Form=Parallel  TimeDomain=Discrete-time  UseExternalTs=off  SampleTime=-1  IntegratorMethod=Forward Euler  FilterMethod=Forward Euler  ControllerParametersSource=external  P=1  I=1  UseKiTs=on  D=0  N=100  UseFilter=on  TunerSelectOption=Transfer Function Based (PID Tuner App)  InitialConditionSource=external  InitialConditionForIntegrator=0  InitialConditionForFilter=0  DifferentiatorICPrevScaledInput=0  ExternalReset=level  TrackingMode=off  Kt=1  LimitOutput=on  SatLimitsSource=internal  UpperSaturationLimit=1  LowerSaturationLimit=-1  LinearizeAsGain=on  AntiWindupMode=clamping  Kb=1  LimitIntegrator=off  UpperIntegratorSaturationLimit=inf  LowerIntegratorSaturationLimit=-inf  RndMeth=Simplest  POutMin=[]  POutMax=[]  IOutMin=[]  IOutMax=[]  DOutMin=[]  DOutMax=[]  NOutMin=[]  NOutMax=[]  SumOutMin=[]  SumOutMax=[]  SaturationOutDataTypeStr=Inherit: Inherit via back propagation  SaturationOutMin=[]  SaturationOutMax=[]  PParamMin=[]  PParamMax=[]  IParamMin=[]  IParamMax=[]  DParamMin=[]  DParamMax=[]  NParamMin=[]  NParamMax=[]  KbParamMin=[]  KbParamMax=[]  KtParamMin=[]  KtParamMax=[]  KbOutMin=[]  KbOutMax=[]  KtOutMin=[]  KtOutMax=[]  IntegratorOutMin=[]  IntegratorOutMax=[]  FilterOutMin=[]  FilterOutMax=[]  SumI1OutMin=[]  SumI1OutMax=[]  SumI2OutMin=[]  SumI2OutMax=[]  SumI3OutMin=[]  SumI3OutMax=[]  SumI4OutMin=[]  SumI4OutMax=[]  SumDOutMin=[]  SumDOutMax=[]  DifferentiatorOutMin=[]  DifferentiatorOutMax=[]  FilterDiffOutCoefMin=[]  FilterDiffOutCoefMax=[]  ReciprocalOutMin=[]  ReciprocalOutMax=[]  SumDenOutMin=[]  SumDenOutMax=[]  SumNumOutMin=[]  SumNumOutMax=[]  DivideOutMin=[]  DivideOutMax=[]  UdiffTsProdOutMin=[]  UdiffTsProdOutMax=[]  NTsProdOutMin=[]  NTsProdOutMax=[]  UintegralTsProdOutMin=[]  UintegralTsProdOutMax=[]  UngainTsProdOutMin=[]  UngainTsProdOutMax=[]  ClampingZeroOutDataTypeStr=Inherit: Inherit via back propagation  ClampingZeroOutMin=[]  ClampingZeroOutMax=[]  FilterDenConstantOutDataTypeStr=Inherit: Inherit via back propagation  FilterDenConstantOutMin=[]  FilterDenConstantOutMax=[]  PCopyOutDataTypeStr=Inherit: Inherit via back propagation  PCopyOutMin=[]  PCopyOutMax=[]  NCopyOutDataTypeStr=Inherit: Inherit via back propagation  NCopyOutMin=[]  NCopyOutMax=[]  IntegratorContinuousStateAttributes=''  IntegratorStateMustResolveToSignalObject=off  IntegratorRTWStateStorageClass=Auto  FilterContinuousStateAttributes=''  FilterStateMustResolveToSignalObject=off  FilterRTWStateStorageClass=Auto  ParallelPVariant=ExternalParameters  IdealPVariant=Disabled  IVariant=ExternalParameters  DVariant=Disabled  IntegratorVariant=Discrete  SatVariant=Enabled  AWVariant=DiscClampingParallel  PCopyVariant=Disabled  TRVariant=Disabled  FdbkBlocksVariant=Forward  IdealPFdbkVariant=Disabled  SatFdbkVariant=Disabled  DerivativeFilterVariant=Disabled  NVariant=Disabled  NCopyVariant=Disabled_SignalSpec  FilterICVariant=Disabled  IntegratorICVariant=ExternalICs  ExternalResetVariant=ExternalReset  TRSumVariant=Passthrough  SumFdbkVariant=Disabled  SumVariant=Sum_PI  TsampFilterVariant=InternalTs  TsampNgainVariant=Passthrough  TsampIntegralVariant=Disabled_SignalSpec  ExternalSaturationOutDataTypeStr=Inherit: Same as second input
      settings: LibrarySourceBlock=mcbcontrolslib/PI Controller
  Ki1 : Constant  Value=PI_params.Ki_speed*Ts_speed  OutDataTypeStr=dataType  SampleTime=-1
  Ki2 : Constant  Value=0  OutDataTypeStr=dataType  SampleTime=-1
  Kp1 : Constant  Value=PI_params.Kp_speed  OutDataTypeStr=dataType  SampleTime=-1
  Logical Operator : Logic  Operator=NOT  IconShape=distinctive  AllPortsSameDT=off  OutDataTypeStr=boolean
  Sum : Sum  Inputs=|+-  RndMeth=Simplest  OutDataTypeStr=Inherit: Same as first input
  Iq_ref : Outport  VectorParamsAs1DForOutWhenUnconnected=off
  wires:
  Discrete PI Controller with anti-windup & reset/1 -> Iq_ref/1
  Ki1/1 -> Discrete PI Controller with anti-windup & reset/3
  Kp1/1 -> Discrete PI Controller with anti-windup & reset/2
  N_fb/1 -> Sum/2
  Sum/1 -> Discrete PI Controller with anti-windup & reset/1
  Ki2/1 -> Discrete PI Controller with anti-windup & reset/5
  Data Store Read1/1 -> Logical Operator/1
  Logical Operator/1 -> Discrete PI Controller with anti-windup & reset/4
  N_ref/1 -> Sum/1

== system mcb_pmsm_foc_hall_f28069m/Speed Control/Speed_Ref_Selector ==
  Speed_Ref_In : Inport
  Speed_Ref_Open : Inport  Port=2
  Data Store Read1 : DataStoreRead  DataStoreName=Enable  IndexOptions=Index vector (dialog)  Indices=1  OutputSizes=1
  IIR Filter : mcbcontrolslib/IIR Filter  VariantControl=Low Pass Filter  VariantSelect=Low-pass  Filter_constant=0.01  advancedSettings=off  Ts=50e-6  cutOff_freq=32.1525
  Switch : Switch  Criteria=u2 > Threshold  Threshold=0.5  SaturateOnIntegerOverflow=off  InputSameDT=off
  Speed_Ref_PU : Outport
  wires:
  IIR Filter/1 -> Speed_Ref_PU/1
  Switch/1 -> IIR Filter/1
  Data Store Read1/1 -> Switch/2
  Speed_Ref_Open/1 -> Switch/3
  Speed_Ref_In/1 -> Switch/1

== system mcb_pmsm_foc_hall_f28069m/Current Control/Control_System/Current_Controllers ==
  Id : Inport
  Iq : Inport  Port=2
  Idq_ref_PU : Inport  Port=3
  DQ Limiter : mcbcontrolslib/DQ Limiter  satMethodInputType=Specify via dialog  satMethodSelected=D-Q equivalence  satLimitInputType=Specify via dialog  Vmax=0.95
  Demux : Demux  Outputs=2
  Mux : Mux
  PI_Controller_Id : Subsystem
  PI_Controller_Iq : Subsystem
  Terminator : Terminator
  Vd_ref : Outport  VectorParamsAs1DForOutWhenUnconnected=off
  Vq_ref : Outport  Port=2  VectorParamsAs1DForOutWhenUnconnected=off
  Idq : Outport  Port=3  VectorParamsAs1DForOutWhenUnconnected=off
  wires:
  Iq/1 -> Mux/4, PI_Controller_Iq/2(I_fb)  "Iq_fb"
  Id/1 -> Mux/2, PI_Controller_Id/2(I_fb)  "Id_fb"
  Demux/1 -> Mux/1, PI_Controller_Id/1(I_ref)  "Id_Ref"
  Demux/2 -> Mux/3, PI_Controller_Iq/1(I_ref)  "Iq_Ref"
  PI_Controller_Id/1(V_ref) -> DQ Limiter/1
  PI_Controller_Iq/1(V_ref) -> DQ Limiter/2
  Idq_ref_PU/1 -> Demux/1
  DQ Limiter/2 -> Vq_ref/1
  DQ Limiter/1 -> Vd_ref/1
  DQ Limiter/3 -> Terminator/1
  Mux/1 -> Idq/1

== system mcb_pmsm_foc_hall_f28069m/Current Control/Data_Logging/Data ==
  Data : Inport
  Data_width : Inport  Port=2
  Action Port : ActionPort  ActionPortLabel=else
  Mux : Mux  Inputs=2
  Start : Constant  Value=hex2dec('0000')  OutDataTypeStr=uint16
  Data_out : Outport  VectorParamsAs1DForOutWhenUnconnected=off
  Iteration : Outport  Port=2  VectorParamsAs1DForOutWhenUnconnected=off
  wires:
  Start/1 -> Mux/2
  Mux/1 -> Data_out/1
  Data/1 -> Mux/1
  Data_width/1 -> Iteration/1

== system mcb_pmsm_foc_hall_f28069m/Current Control/Data_Logging/Data_Conditioning ==
  In1 : Inport
  Data Type Conversion : DataTypeConversion  OutDataTypeStr=fixdt(1,32,12)  RndMeth=Simplest  SaturateOnIntegerOverflow=off
  Data Type Conversion3 : DataTypeConversion  OutDataTypeStr=uint16  ConvertRealWorld=Stored Integer (SI)  RndMeth=Simplest  SaturateOnIntegerOverflow=off
  Out1 : Outport  VectorParamsAs1DForOutWhenUnconnected=off
  wires:
  In1/1 -> Data Type Conversion/1
  Data Type Conversion3/1 -> Out1/1
  Data Type Conversion/1 -> Data Type Conversion3/1

== system mcb_pmsm_foc_hall_f28069m/Current Control/Data_Logging/End ==
  Data : Inport
  Data_width : Inport  Port=2
  Action Port : ActionPort  ActionPortLabel=elseif(u1 == 599)
  Bias : Bias  Bias=1  SaturateOnIntegerOverflow=off
  Mux : Mux  Inputs=2
  Start : Constant  Value=hex2dec('4545')  OutDataTypeStr=uint16
  Data_out : Outport  VectorParamsAs1DForOutWhenUnconnected=off
  Iteration : Outport  Port=2  VectorParamsAs1DForOutWhenUnconnected=off
  wires:
  Mux/1 -> Data_out/1
  Data_width/1 -> Bias/1
  Start/1 -> Mux/2
  Bias/1 -> Iteration/1
  Data/1 -> Mux/1

== system mcb_pmsm_foc_hall_f28069m/Current Control/Data_Logging/Start ==
  Data : Inport
  Data_width : Inport  Port=2
  Action Port : ActionPort  ActionPortLabel=if(u1 == 0)
  Bias : Bias  Bias=1  SaturateOnIntegerOverflow=off
  End : Constant  Value=hex2dec('5353')  OutDataTypeStr=uint16
  Mux : Mux  Inputs=2
  Data_out : Outport  VectorParamsAs1DForOutWhenUnconnected=off
  Iteration : Outport  Port=2  VectorParamsAs1DForOutWhenUnconnected=off
  wires:
  End/1 -> Mux/1
  Mux/1 -> Data_out/1
  Data_width/1 -> Bias/1
  Bias/1 -> Iteration/1
  Data/1 -> Mux/2

== system mcb_pmsm_foc_hall_f28069m/Current Control/Input Scaling/Read_Sensor (codegen) ==
  Iab_meas_ADC : Inport  OutDataTypeStr=uint16
  Iab_Sim : Inport  Port=2
  Pos_Sim : Inport  Port=3
  Calculate Position from Hall : Subsystem
  Convert ADC value to PU : Subsystem
  Terminator : Terminator
  Terminator1 : Terminator
  Iab_Meas_PU : Outport  VectorParamsAs1DForOutWhenUnconnected=off
  Pos_PU : Outport  Port=2  VectorParamsAs1DForOutWhenUnconnected=off
  Speed_PU : Outport  Port=3  VectorParamsAs1DForOutWhenUnconnected=off
  wires:
  Iab_Sim/1 -> Terminator/1
  Calculate Position from Hall/1(Pos_PU) -> Pos_PU/1
  Iab_meas_ADC/1 -> Convert ADC value to PU/1(Iab_meas_ADC)
  Convert ADC value to PU/1(Iab_meas_PU) -> Iab_Meas_PU/1
  Pos_Sim/1 -> Terminator1/1
  Calculate Position from Hall/2(Speed_PU) -> Speed_PU/1

== system mcb_pmsm_foc_hall_f28069m/Current Control/Input Scaling/Read_Sensor (sim) ==
  Iab_meas_ADC : Inport
  Iab_Sim : Inport  Port=2
  Pos_Sim : Inport  Port=3
  Convert ADC value to PU : Subsystem
  Subsystem : Subsystem
  Terminator : Terminator
  Iab_Meas_PU : Outport  VectorParamsAs1DForOutWhenUnconnected=off
  Pos_PU : Outport  Port=2  VectorParamsAs1DForOutWhenUnconnected=off
  Speed_PU : Outport  Port=3  VectorParamsAs1DForOutWhenUnconnected=off
  wires:
  Iab_meas_ADC/1 -> Terminator/1
  Iab_Sim/1 -> Convert ADC value to PU/1(Iab_meas_ADC)
  Convert ADC value to PU/1(Iab_meas_PU) -> Iab_Meas_PU/1
  Pos_Sim/1 -> Subsystem/1(Pos_Sim)
  Subsystem/1(Theta) -> Pos_PU/1
  Subsystem/2(Speed) -> Speed_PU/1
